simulink model "gps_subscription"  (R2020a)
settings: Solver=VariableStepAuto  StartTime=0.0  StopTime=inf  RelTol=1e-3
libraries: robotlib x2, robotcorelib x1
settings Model: Creator=root  LastModifiedBy=root

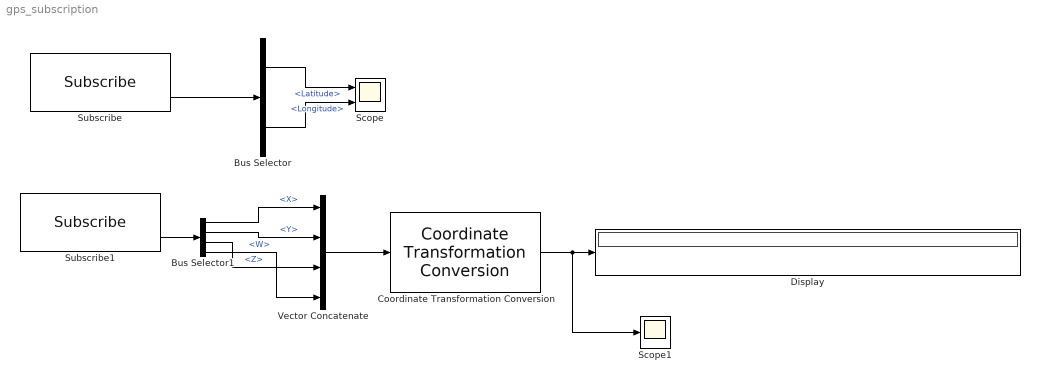
== system gps_subscription ==
  Bus Selector : BusSelector  OutputSignals=Latitude,Longitude
  Bus Selector1 : BusSelector  OutputSignals=Pose.Pose.Orientation.X,Pose.Pose.Orientation.Y,Pose.Pose.Orientation.Z,Pose.Pose.Orientation.W
  Coordinate Transformation Conversion : robotcorelib/Coordinate Transformation Conversion  InputRepresentation=Quaternion  InputEulerSequence=ZYX  ShowTrVecInputPort=on  OutputRepresentation=Euler Angles  OutputEulerSequence=XYZ  ShowTrVecOutputPort=on  SimulateUsing=Interpreted execution
      settings: SourceProductBaseCode=NV,RO,RR
  Display : Display
  Scope : Scope  NumInputPorts=2
  Scope1 : Scope
  Subscribe : robotlib/Subscribe  topicSource=Select from ROS network  topic=/gps_lat_long  messageType=gps_msgs/gps  sampleTime=-1  messageQueueLength=1
  Subscribe1 : robotlib/Subscribe  topicSource=Select from ROS network  topic=/odom  messageType=nav_msgs/Odometry  sampleTime=-1  messageQueueLength=1
  Vector Concatenate : Concatenate  NumInputs=4
  wires:
  Subscribe/2 -> Bus Selector/1
  Bus Selector/1 -> Scope/1  "<Latitude>"
  Bus Selector/2 -> Scope/2  "<Longitude>"
  Subscribe1/2 -> Bus Selector1/1
  Bus Selector1/1 -> Vector Concatenate/1  "<X>"
  Bus Selector1/2 -> Vector Concatenate/2  "<Y>"
  Bus Selector1/3 -> Vector Concatenate/3  "<Z>"
  Bus Selector1/4 -> Vector Concatenate/4  "<W>"
  Vector Concatenate/1 -> Coordinate Transformation Conversion/1
  Coordinate Transformation Conversion/1 -> Scope1/1, Display/1
